simulink model "dynsim_3link_planar"  (R2020a)
settings: Solver=FixedStepAuto  StartTime=0.0  StopTime=10.0  FixedStep=0.001  RelTol=1e-3
values from neighbouring files (symbols this model uses):
  L1 = 1    [init_3link_planar.m]
  L2 = 1    [init_3link_planar.m]
  L3 = 1    [init_3link_planar.m]
libraries: robotlib x12, robotmaniplib x1
settings Model: Creator=bascetta  LastModifiedBy=cesare
settings OptimizationCC: EnhancedBackFolding=on  PassReuseOutputArgsAs=Individual arguments  ZeroExternalMemoryAtStartup=off  ZeroInternalMemoryAtStartup=off  MaxStackSize=64  OptimizeBlockOrder=speed  DifferentSizesBufferReuse=on  OptimizationCustomize=off  EfficientTunableParamExpr=on
settings DebuggingCC: ParameterTunabilityLossMsg=error
settings HardwareCC: ProdBitPerPointer=32  ProdBitPerSizeT=32  ProdBitPerPtrDiffT=32  ProdLargestAtomicFloat=None  ProdIntDivRoundTo=Undefined  ProdEndianess=Unspecified  ProdWordSize=32  ProdHWDeviceType=Generic->Unspecified (assume 32-bit Generic)  UseEmbeddedCoderFeatures=off
settings RTWCC: SystemTargetFile=ert.tlc  HardwareBoard=Robot Operating System (ROS)  TemplateMakefile=ert_default_tmf  GenerateReport=on  Toolchain=Catkin  IncludeHyperlinkInReport=on  LaunchReport=on  TargetLang=C++  GenerateTraceInfo=on  GenerateTraceReport=on  GenerateTraceReportSl=on  GenerateTraceReportSf=on  GenerateTraceReportEml=on
settings CodeAppCC: ForceParamTrailComments=on  IgnoreCustomStorageClasses=off  OperatorAnnotations=on  SimulinkDataObjDesc=on  SFDataObjDesc=on  InsertBlockDesc=on
settings ERTTargetCC: SupportContinuousTime=on  SupportNonInlinedSFcns=on  SupportVariableSizeSignals=on

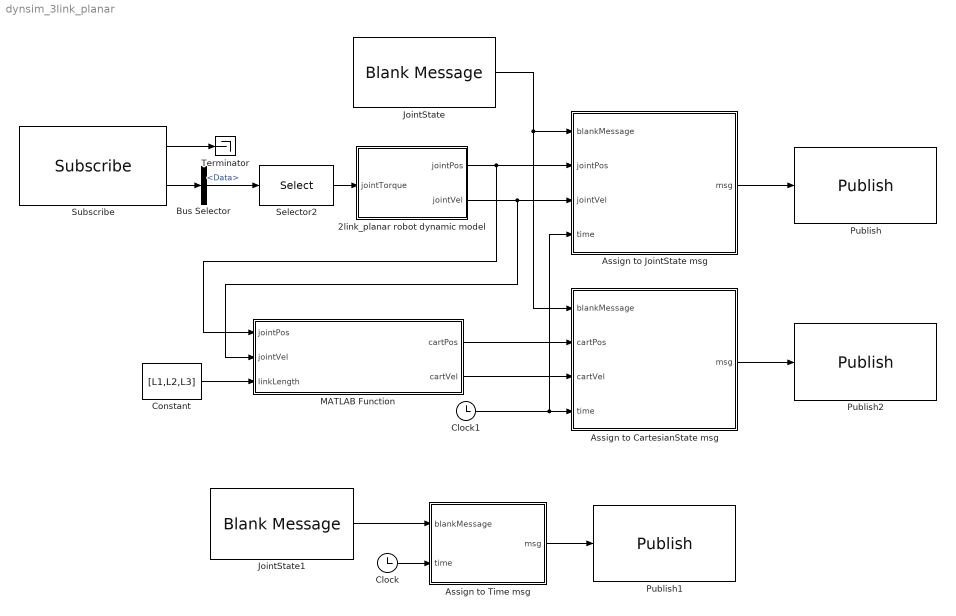
== system dynsim_3link_planar ==
  2link_planar robot dynamic model : Subsystem
  Assign to CartesianState msg : MATLAB Function  TreatAsAtomicUnit=on
  Assign to JointState msg : MATLAB Function  TreatAsAtomicUnit=on
  Assign to Time msg : MATLAB Function  TreatAsAtomicUnit=on
  Bus Selector : BusSelector  OutputSignals=Data
  Clock : Clock
  Clock1 : Clock
  Constant : Constant  Value=[L1,L2,L3]
  JointState : robotlib/Blank Message  messageClass=Message  entityType=sensor_msgs/JointState  messageType=sensor_msgs/JointState  SampleTime=inf
  JointState1 : robotlib/Blank Message  messageClass=Message  entityType=rosgraph_msgs/Clock  messageType=rosgraph_msgs/Clock  SampleTime=inf
  MATLAB Function : MATLAB Function  TreatAsAtomicUnit=on
  Publish : robotlib/Publish  topicSource=Specify your own  topic=/joint_states  messageType=sensor_msgs/JointState  messageQueueLength=1
  Publish1 : robotlib/Publish  topicSource=Specify your own  topic=/clock  messageType=rosgraph_msgs/Clock  messageQueueLength=1
  Publish2 : robotlib/Publish  topicSource=Specify your own  topic=/cartesian_states  messageType=sensor_msgs/JointState  messageQueueLength=1
  Selector2 : Selector  IndexOptions=Starting index (dialog)  Indices=[2]  OutputSizes=3
  Subscribe : robotlib/Subscribe  topicSource=Specify your own  topic=/joint_torque  messageType=std_msgs/Float64MultiArray  sampleTime=-1  messageQueueLength=1
  Terminator : Terminator
  wires:
  JointState1/1 -> Assign to Time msg/1(blankMessage)
  Assign to Time msg/1(msg) -> Publish1/1
  Subscribe/2 -> Bus Selector/1
  Subscribe/1 -> Terminator/1
  Selector2/1 -> 2link_planar robot dynamic model/1(jointTorque)
  Assign to JointState msg/1(msg) -> Publish/1
  2link_planar robot dynamic model/2(jointVel) -> MATLAB Function/2(jointVel), Assign to JointState msg/3(jointVel)
  Bus Selector/1 -> Selector2/1  "<Data>"
  2link_planar robot dynamic model/1(jointPos) -> MATLAB Function/1(jointPos), Assign to JointState msg/2(jointPos)
  Clock/1 -> Assign to Time msg/2(time)
  Clock1/1 -> Assign to CartesianState msg/4(time), Assign to JointState msg/4(time)
  MATLAB Function/2(cartVel) -> Assign to CartesianState msg/3(cartVel)
  Assign to CartesianState msg/1(msg) -> Publish2/1
  Constant/1 -> MATLAB Function/3(linkLength)
  MATLAB Function/1(cartPos) -> Assign to CartesianState msg/2(cartPos)
  JointState/1 -> Assign to CartesianState msg/1(blankMessage), Assign to JointState msg/1(blankMessage)

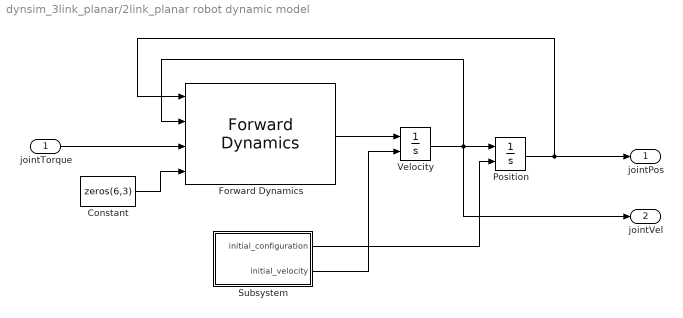
== system dynsim_3link_planar/2link_planar robot dynamic model ==
  jointTorque : Inport
  Constant : Constant  Value=zeros(6,3)
  Forward Dynamics : robotmaniplib/Forward Dynamics  RigidBodyTree=robot_3link_planar  SimulateUsing=Interpreted execution
  Position : Integrator  InitialConditionSource=external
  Subsystem : Subsystem
  Velocity : Integrator  InitialConditionSource=external
  jointPos : Outport
  jointVel : Outport  Port=2
  wires:
  Forward Dynamics/1 -> Velocity/1
  Position/1 -> Forward Dynamics/1, jointPos/1
  jointTorque/1 -> Forward Dynamics/3
  Constant/1 -> Forward Dynamics/4
  Velocity/1 -> Forward Dynamics/2, Position/1, jointVel/1
  Subsystem/2(initial_velocity) -> Velocity/2
  Subsystem/1(initial_configuration) -> Position/2

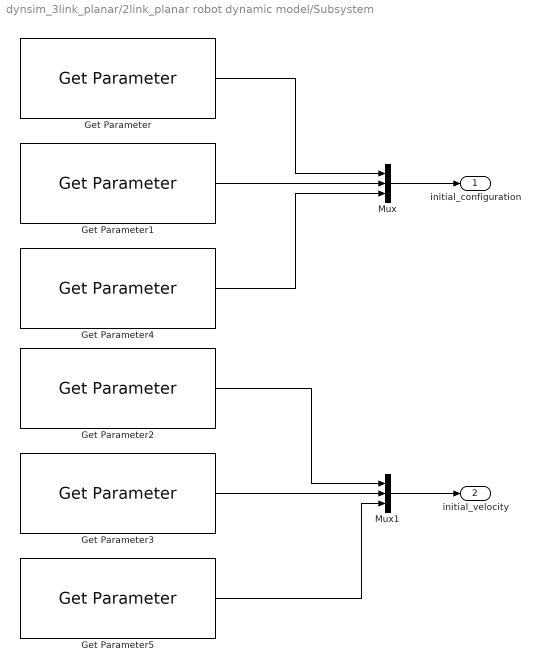
== system dynsim_3link_planar/2link_planar robot dynamic model/Subsystem ==
  Get Parameter : robotlib/Get Parameter  ParameterSource=Specify your own  ParameterName=/dynsim_3link_planar/q1_initial  ParameterType=double  ParameterMaxArrayLength=16  ParameterInitialValue=pi/4  SampleTime=-1  ShowErrorCodeOutput=off  ModelName=dynsim_3link_planar  BlockId=ParamGet_dynsim_3link_planar_112
      settings: SourceProductBaseCode=RR
  Get Parameter1 : robotlib/Get Parameter  ParameterSource=Specify your own  ParameterName=/dynsim_3link_planar/q2_initial  ParameterType=double  ParameterMaxArrayLength=16  ParameterInitialValue=-pi/2  SampleTime=-1  ShowErrorCodeOutput=off  ModelName=dynsim_3link_planar  BlockId=ParamGet_dynsim_3link_planar_113
      settings: SourceProductBaseCode=RR
  Get Parameter2 : robotlib/Get Parameter  ParameterSource=Specify your own  ParameterName=/dynsim_3link_planar/qv1_initial  ParameterType=double  ParameterMaxArrayLength=16  ParameterInitialValue=0  SampleTime=-1  ShowErrorCodeOutput=off  ModelName=dynsim_3link_planar  BlockId=ParamGet_dynsim_3link_planar_117
      settings: SourceProductBaseCode=RR
  Get Parameter3 : robotlib/Get Parameter  ParameterSource=Specify your own  ParameterName=/dynnsim_3link_planar/qv2_initial  ParameterType=double  ParameterMaxArrayLength=16  ParameterInitialValue=0  SampleTime=-1  ShowErrorCodeOutput=off  ModelName=dynsim_3link_planar  BlockId=ParamGet_dynsim_3link_planar_118
      settings: SourceProductBaseCode=RR
  Get Parameter4 : robotlib/Get Parameter  ParameterSource=Specify your own  ParameterName=/dynsim_3link_planar/q3_initial  ParameterType=double  ParameterMaxArrayLength=16  ParameterInitialValue=0  SampleTime=-1  ShowErrorCodeOutput=off  ModelName=dynsim_3link_planar  BlockId=ParamGet_dynsim_3link_planar_125
      settings: SourceProductBaseCode=RR
  Get Parameter5 : robotlib/Get Parameter  ParameterSource=Specify your own  ParameterName=/dynnsim_3link_planar/qv3_initial  ParameterType=double  ParameterMaxArrayLength=16  ParameterInitialValue=0  SampleTime=-1  ShowErrorCodeOutput=off  ModelName=dynsim_3link_planar  BlockId=ParamGet_dynsim_3link_planar_126
      settings: SourceProductBaseCode=RR
  Mux : Mux  Inputs=3
  Mux1 : Mux  Inputs=3
  initial_configuration : Outport
  initial_velocity : Outport  Port=2
  wires:
  Mux/1 -> initial_configuration/1
  Get Parameter/1 -> Mux/1
  Get Parameter1/1 -> Mux/2
  Get Parameter3/1 -> Mux1/2
  Get Parameter2/1 -> Mux1/1
  Mux1/1 -> initial_velocity/1
  Get Parameter4/1 -> Mux/3
  Get Parameter5/1 -> Mux1/3

== matlab function dynsim_3link_planar/Assign to Time msg ==
  data: blankMessage input; msg output Bus: SL_Bus_dynsim_3link_planar_rosgraph_msgs_Clock; time input
function msg = assign_Time(blankMessage,time)
%#codegen

% Assign the output message to be the same with input blank message
msg = blankMessage;

% Convert and set time
msg.Clock_.Sec  = fix(time);
msg.Clock_.Nsec = fix((time-fix(time))*1e9);

== matlab function dynsim_3link_planar/Assign to JointState msg ==
  data: blankMessage input; msg output Bus: SL_Bus_dynsim_3link_planar_sensor_msgs_JointState; jointPos input; jointVel input; time input
function msg = assign_JointState(blankMessage,jointPos,jointVel,time)
%#codegen

% Assign the output message to be the same with input blank message
msg = blankMessage;

% Initialize time stamp
msg.Header.Stamp.Sec  = fix(time);
msg.Header.Stamp.Nsec = fix((time-fix(time))*1e9);

% Set the number of strings in the string array, and joint positions/velocities in the position/velocity array
numJoints = length(jointPos);
msg.Name_SL_Info.CurrentLength = uint32(numJoints);
msg.Position_SL_Info.CurrentLength = uint32(numJoints);
msg.Velocity_SL_Info.CurrentLength = uint32(numJoints);

% Set the individual components in the message arrays
strArrayToAssign = {'arm_joint', 'forearm_joint','wrist_joint'};

for idx=1:numJoints
    str = strArrayToAssign{idx};
    strLength = length(str);
    msg.Name(idx).Data(1:strLength) = uint8(str);
    msg.Name(idx).Data_SL_Info.CurrentLength = uint32(strLength);

    msg.Position(idx) = jointPos(idx);
    msg.Velocity(idx) = jointVel(idx);
end

== matlab function dynsim_3link_planar/MATLAB Function ==
  data: jointPos input; cartPos output; jointVel input; cartVel output; linkLength input
function [cartPos, cartVel] = forward_kinematics_3link(jointPos,jointVel,linkLength)

cartPos = zeros(1,2);
cartVel = zeros(1,2);

L1 = linkLength(1);
L2 = linkLength(2);
L3 = linkLength(3);
q1 = jointPos(1);
q2 = jointPos(2);
q3 = jointPos(3);
qv1 = jointVel(1);
qv2 = jointVel(2);
qv3 = jointVel(3);

cartPos(1) = L1*cos(q1)+L2*cos(q1+q2)+L3*cos(q1+q2+q3);
cartPos(2) = L1*sin(q1)+L2*sin(q1+q2)+L3*sin(q1+q2+q3);
cartVel(1) = -L1*qv1*sin(q1)-L2*(qv1+qv2)*sin(q1+q2)-L3*(qv1+qv2+qv3)*sin(q1+q2+q3);
cartVel(2) = L1*qv1*cos(q1)+L2*(qv1+qv2)*cos(q1+q2)+L3*(qv1+qv2+qv3)*cos(q1+q2+q3);

== matlab function dynsim_3link_planar/Assign to CartesianState msg ==
  data: blankMessage input; msg output Bus: SL_Bus_dynsim_3link_planar_sensor_msgs_JointState; cartPos input; cartVel input; time input
function msg = assign_CartesianState(blankMessage,cartPos,cartVel,time)
%#codegen

% Assign the output message to be the same with input blank message
msg = blankMessage;

% Initialize time stamp
msg.Header.Stamp.Sec  = fix(time);
msg.Header.Stamp.Nsec = fix((time-fix(time))*1e9);

% Set the number of strings in the string array, and joint positions/velocities in the position/velocity array
numCoordinates = length(cartPos);
msg.Name_SL_Info.CurrentLength = uint32(numCoordinates);
msg.Position_SL_Info.CurrentLength = uint32(numCoordinates);
msg.Velocity_SL_Info.CurrentLength = uint32(numCoordinates);

% Set the individual components in the message arrays
strArrayToAssign = {'arm_joint', 'forearm_joint','wrist_joint'};

for idx=1:numCoordinates
    str = strArrayToAssign{idx};
    strLength = length(str);
    msg.Name(idx).Data(1:strLength) = uint8(str);
    msg.Name(idx).Data_SL_Info.CurrentLength = uint32(strLength);

    msg.Position(idx) = cartPos(idx);
    msg.Velocity(idx) = cartVel(idx);
end
